simulink model "samp"  (R2012b)
settings: Solver=FixedStepDiscrete  StartTime=0.0  StopTime=1  FixedStep=dt  RelTol=1e-3
InitFcn:
  | param
values from neighbouring files (symbols this model uses):
  ampl = 5    [param.m]
  dt = 0.00005    (= 5e-05)    [param.m]
  freq = 5000    [param.m]
  noiseVariance = 10    [param.m]
  T = 0.15    [param.m]
undefined symbols (not defined in the file or in its folder): DiscIntNeverNeededParam
libraries: commchan3 x1
settings Model: Creator=mishuk  LastModifiedBy=mishuk

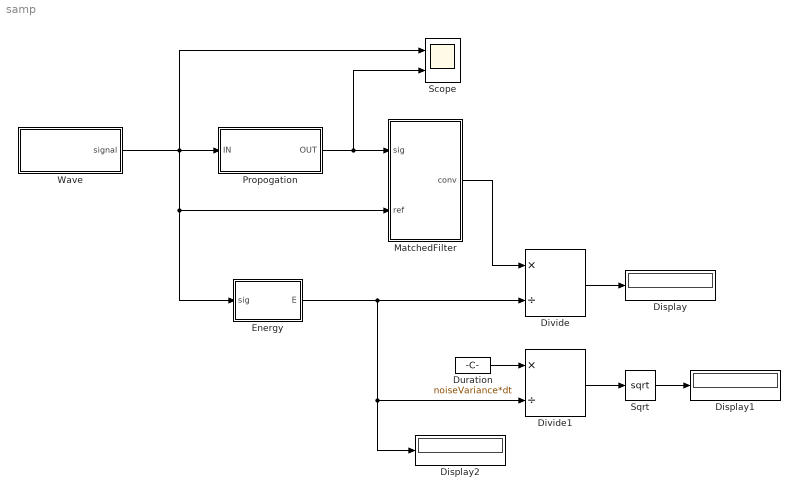
== system samp ==
  Display : Display
  Display1 : Display
  Display2 : Display
  Divide : Product  Inputs=*/
  Divide1 : Product  Inputs=*/
  Duration : Constant  Value=noiseVariance*dt
  Energy : Subsystem
  MatchedFilter : Subsystem
  Propogation : Subsystem
  Scope : Scope  NumInputPorts=2
      settings: TimeRange=1  YMin=-1~-4  YMax=1~6
  Sqrt : Sqrt  SaturateOnIntegerOverflow=on
  Wave : Subsystem
  wires:
  Wave/1(signal) -> Scope/1, Energy/1(sig), MatchedFilter/2(ref), Propogation/1(IN)
  Propogation/1(OUT) -> Scope/2, MatchedFilter/1(sig)
  MatchedFilter/1(conv) -> Divide/1
  Energy/1(E) -> Display2/1, Divide1/2, Divide/2
  Divide/1 -> Display/1
  Duration/1 -> Divide1/1
  Divide1/1 -> Sqrt/1
  Sqrt/1 -> Display1/1

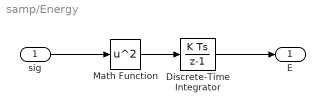
== system samp/Energy ==
  sig : Inport
  Discrete-Time Integrator : DiscreteIntegrator  InitialCondition=1e-10  SampleTime=dt  ICPrevOutput=DiscIntNeverNeededParam  ICPrevScaledInput=DiscIntNeverNeededParam
  Math Function : Math  Operator=square  SaturateOnIntegerOverflow=on
  E : Outport
  wires:
  Discrete-Time Integrator/1 -> E/1
  sig/1 -> Math Function/1
  Math Function/1 -> Discrete-Time Integrator/1

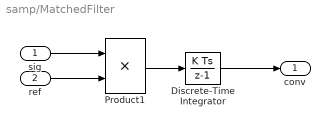
== system samp/MatchedFilter ==
  sig : Inport
  ref : Inport  Port=2
  Discrete-Time Integrator : DiscreteIntegrator  SampleTime=dt  ICPrevOutput=DiscIntNeverNeededParam  ICPrevScaledInput=DiscIntNeverNeededParam
  Product1 : Product  RndMeth=Zero
  conv : Outport
  wires:
  Product1/1 -> Discrete-Time Integrator/1
  ref/1 -> Product1/2
  sig/1 -> Product1/1
  Discrete-Time Integrator/1 -> conv/1

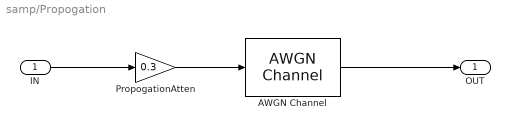
== system samp/Propogation ==
  IN : Inport
  AWGN Channel : commchan3/AWGN Channel  InputProcessing=Columns as channels (frame based)  seed=67  noiseMode=Variance from mask  EbNodB=10  EsNodB=10  SNRdB=0  bitsPerSym=1  Ps=0.01  Tsym=1  variance=noiseVariance
  PropogationAtten : Gain  Gain=0.3
  OUT : Outport
  wires:
  PropogationAtten/1 -> AWGN Channel/1
  IN/1 -> PropogationAtten/1
  AWGN Channel/1 -> OUT/1

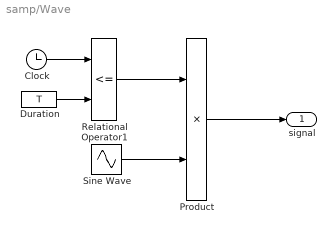
== system samp/Wave ==
  Clock : Clock
  Duration : Constant  Value=T
  Product : Product  RndMeth=Zero
  Relational Operator1 : RelationalOperator  Operator=<=  OutDataTypeStr=boolean
  Sine Wave : Sin  Amplitude=ampl  Frequency=2*pi*freq  Phase=2*pi*rand(1)  SampleTime=dt
  signal : Outport
  wires:
  Duration/1 -> Relational Operator1/2
  Product/1 -> signal/1
  Clock/1 -> Relational Operator1/1
  Sine Wave/1 -> Product/2
  Relational Operator1/1 -> Product/1
